simulink model "cesna_a_37_impl"  (Simulink 7.5)
settings: Solver=ode45  StartTime=0.0  StopTime=200  RelTol=1e-3
undefined symbols (not defined in the file): A, alpha_trim, B, C, D, F_T_trim
libraries: simulink x3, Airframes x1
(part 2 of 2)

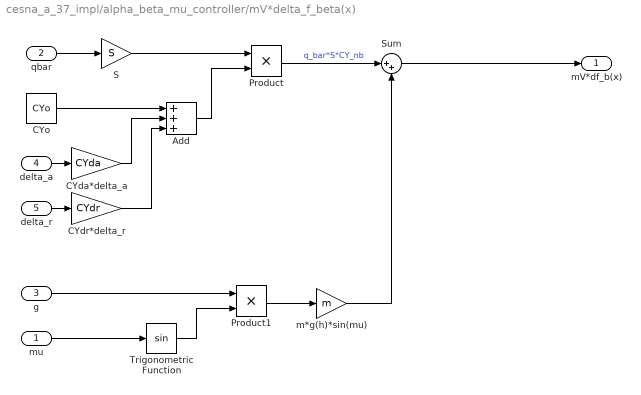
== system cesna_a_37_impl/alpha_beta_mu_controller/mV*delta_f_beta(x) ==
  mu : Inport  OutDataType=fixdt(1, 16)  OutScaling=2^0
  qbar : Inport  Port=2  OutDataType=fixdt(1, 16)  OutScaling=2^0
  g : Inport  Port=3  OutDataType=fixdt(1, 16)  OutScaling=2^0
  delta_a : Inport  Port=4  OutDataType=fixdt(1, 16)  OutScaling=2^0
  delta_r : Inport  Port=5  OutDataType=fixdt(1, 16)  OutScaling=2^0
  Add : Sum  Inputs=+++  OutDataType=fixdt(1, 16)  OutScaling=2^-10
  CYda*delta_a : Gain  Gain=CYda  ParameterDataTypeMode=single  ParameterDataType=fixdt(1, 16)  ParameterScaling=2^0  ParamDataTypeStr=single  OutDataType=fixdt(1, 16)  OutScaling=2^0
  CYdr*delta_r : Gain  Gain=CYdr  ParameterDataTypeMode=single  ParameterDataType=fixdt(1, 16)  ParameterScaling=2^0  ParamDataTypeStr=single  OutDataType=fixdt(1, 16)  OutScaling=2^0
  CYo : Constant  Value=CYo  OutDataTypeMode=single  OutDataType=fixdt(1, 16)  OutScaling=2^0  OutDataTypeStr=single
  Product : Product  OutDataType=fixdt(1, 16)  OutScaling=2^0  RndMeth=Zero
  Product1 : Product  OutDataType=fixdt(1, 16)  OutScaling=2^0  RndMeth=Zero
  S : Gain  Gain=S  ParameterDataTypeMode=single  ParameterDataType=fixdt(1, 16)  ParameterScaling=2^0  ParamDataTypeStr=single  OutDataType=fixdt(1, 16)  OutScaling=2^0
  Sum : Sum  Inputs=|++  OutDataType=fixdt(1, 16)  OutScaling=2^0
  Trigonometric Function : Trigonometry
  m*g(h)*sin(mu) : Gain  Gain=m  ParameterDataTypeMode=single  ParameterDataType=fixdt(1, 16)  ParameterScaling=2^0  ParamDataTypeStr=single  OutDataType=fixdt(1, 16)  OutScaling=2^0
  mV*df_b(x) : Outport  OutDataType=fixdt(1, 16)  OutScaling=2^0
  wires:
  Sum/1 -> mV*df_b(x)/1
  m*g(h)*sin(mu)/1 -> Sum/2
  Product1/1 -> m*g(h)*sin(mu)/1
  Trigonometric Function/1 -> Product1/2
  mu/1 -> Trigonometric Function/1
  g/1 -> Product1/1
  Product/1 -> Sum/1  "q_bar*S*CY_nb"
  CYdr*delta_r/1 -> Add/3
  delta_r/1 -> CYdr*delta_r/1
  delta_a/1 -> CYda*delta_a/1
  CYda*delta_a/1 -> Add/2
  CYo/1 -> Add/1
  Add/1 -> Product/2
  S/1 -> Product/1
  qbar/1 -> S/1

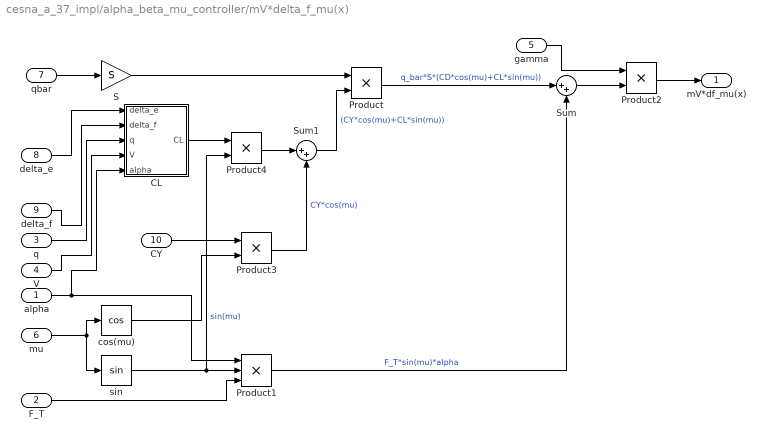
== system cesna_a_37_impl/alpha_beta_mu_controller/mV*delta_f_mu(x) ==
  alpha : Inport  OutDataType=fixdt(1, 16)  OutScaling=2^0
  F_T : Inport  Port=2  OutDataType=fixdt(1, 16)  OutScaling=2^0
  q : Inport  Port=3  OutDataType=fixdt(1, 16)  OutScaling=2^0
  V : Inport  Port=4  OutDataType=fixdt(1, 16)  OutScaling=2^0
  gamma : Inport  Port=5  OutDataType=fixdt(1, 16)  OutScaling=2^0
  mu : Inport  Port=6  OutDataType=fixdt(1, 16)  OutScaling=2^0
  qbar : Inport  Port=7  OutDataType=fixdt(1, 16)  OutScaling=2^0
  delta_e : Inport  Port=8  OutDataType=fixdt(1, 16)  OutScaling=2^0
  delta_f : Inport  Port=9  OutDataType=fixdt(1, 16)  OutScaling=2^0
  CY : Inport  Port=10  OutDataType=fixdt(1, 16)  OutScaling=2^0
  CL : Subsystem
  Product{,2..4} (4 alike) : Product  OutDataType=fixdt(1, 16)  OutScaling=2^0  RndMeth=Zero
  Product1 : Product  Inputs=3  OutDataType=fixdt(1, 16)  OutScaling=2^0  RndMeth=Zero
  S : Gain  Gain=S  ParameterDataTypeMode=single  ParameterDataType=fixdt(1, 16)  ParameterScaling=2^0  ParamDataTypeStr=single  OutDataType=fixdt(1, 16)  OutScaling=2^0
  Sum : Sum  Inputs=|++  OutDataType=fixdt(1, 16)  OutScaling=2^0
  Sum1 : Sum  Inputs=|++  OutDataType=fixdt(1, 16)  OutScaling=2^0
  cos(mu) : Trigonometry  Operator=cos
  sin : Trigonometry
  mV*df_mu(x) : Outport  OutDataType=fixdt(1, 16)  OutScaling=2^0
  wires:
  qbar/1 -> S/1
  S/1 -> Product/1
  Product/1 -> Sum/1  "q_bar*S*(CD*cos(mu)+CL*sin(mu))"
  mu/1 -> sin/1, cos(mu)/1
  Product1/1 -> Sum/2  "F_T*sin(mu)*alpha"
  gamma/1 -> Product2/1
  Sum/1 -> Product2/2
  Product2/1 -> mV*df_mu(x)/1
  F_T/1 -> Product1/3
  sin/1 -> Product1/2, Product4/2  "sin(mu)"
  alpha/1 -> Product1/1, CL/5(alpha)
  delta_f/1 -> CL/2(delta_f)
  delta_e/1 -> CL/1(delta_e)
  Product3/1 -> Sum1/2  "CY*cos(mu)"
  cos(mu)/1 -> Product3/2
  Sum1/1 -> Product/2  "(CY*cos(mu)+CL*sin(mu))"
  q/1 -> CL/3(q)
  V/1 -> CL/4(V)
  CL/1(CL) -> Product4/1
  Product4/1 -> Sum1/1
  CY/1 -> Product3/1

== system cesna_a_37_impl/alpha_beta_mu_controller/sat ==
  mu_set : Inport
  alpha_set : Inport  Port=2
  beta_set : Inport  Port=3
  Mux1 : Mux  Inputs=3
  Saturation1 : Saturate  UpperLimit=pi/4  LowerLimit=-pi/4  OutDataType=fixdt(1, 16)  OutScaling=2^0
  Saturation2 : Saturate  UpperLimit=pi/4  LowerLimit=-pi/4  OutDataType=fixdt(1, 16)  OutScaling=2^0
  Saturation3 : Saturate  UpperLimit=pi/20  LowerLimit=-pi/20  OutDataType=fixdt(1, 16)  OutScaling=2^0
  x_2 : Outport
  wires:
  Mux1/1 -> x_2/1
  mu_set/1 -> Saturation1/1
  alpha_set/1 -> Saturation2/1
  beta_set/1 -> Saturation3/1
  Saturation1/1 -> Mux1/1
  Saturation2/1 -> Mux1/2
  Saturation3/1 -> Mux1/3

== system cesna_a_37_impl/gamma_chi_controller/Calc_CL ==
  alpha : Inport  OutDataType=fixdt(1, 16)  OutScaling=2^0
  delta : Inport  Port=2  OutDataType=fixdt(1, 16)  OutScaling=2^0
  omega : Inport  Port=3  OutDataType=fixdt(1, 16)  OutScaling=2^0
  V : Inport  Port=4  OutDataType=fixdt(1, 16)  OutScaling=2^0
  Add : Sum  Inputs=++++  OutDataType=fixdt(1, 16)  OutScaling=2^-10
  CLa : Gain  Gain=CLa  ParameterDataTypeMode=single  ParameterDataType=fixdt(1, 16)  ParameterScaling=2^0  ParamDataTypeStr=single  OutDataType=fixdt(1, 16)  OutScaling=2^0
  CLo : Constant  Value=CLo  OutDataTypeMode=single  OutDataType=fixdt(1, 16)  OutScaling=2^0  OutDataTypeStr=single
  Divide : Product  Inputs=*/  OutDataType=fixdt(1, 16)  OutScaling=2^-10
  Dot Product : DotProduct  OutDataType=fixdt(1, 16)  OutScaling=2^-10  InputSameDT=on  OutDataTypeStr=Inherit: Inherit via internal rule
  "[CLde,CLin]" : Constant  Value=[CLde,CLin]  OutDataTypeMode=single  OutDataType=fixdt(1, 16)  OutScaling=2^0  OutDataTypeStr=single
  "[q]" : Selector  InputPortWidth=3  IndexOptions=Index vector (dialog)  Indices=[2]  OutputSizes=1
  delta_e,f : Selector  InputPortWidth=4  IndexOptions=Index vector (dialog)  Indices=[1,2]  OutputSizes=1
  q*CLq*cbar/2 : Gain  Gain=CLq*cbar/2  ParameterDataTypeMode=single  ParameterDataType=fixdt(1, 16)  ParameterScaling=2^0  ParamDataTypeStr=single  OutDataType=fixdt(1, 16)  OutScaling=2^0
  CL : Outport  OutDataType=fixdt(1, 16)  OutScaling=2^0
  wires:
  Add/1 -> CL/1
  Divide/1 -> Add/4
  Dot Product/1 -> Add/3
  CLa/1 -> Add/2
  CLo/1 -> Add/1
  V/1 -> Divide/2
  q*CLq*cbar/2/1 -> Divide/1
  alpha/1 -> CLa/1
  "[q]"/1 -> q*CLq*cbar/2/1
  "[CLde,CLin]"/1 -> Dot Product/1
  delta_e,f/1 -> Dot Product/2
  delta/1 -> delta_e,f/1
  omega/1 -> "[q]"/1

== system cesna_a_37_impl/gamma_chi_controller/Calc_CY ==
  beta : Inport  OutDataType=fixdt(1, 16)  OutScaling=2^0
  delta : Inport  Port=2  OutDataType=fixdt(1, 16)  OutScaling=2^0
  omega : Inport  Port=3  OutDataType=fixdt(1, 16)  OutScaling=2^0
  V : Inport  Port=4  OutDataType=fixdt(1, 16)  OutScaling=2^0
  Add : Sum  Inputs=++++  OutDataType=fixdt(1, 16)  OutScaling=2^-10
  CYb : Gain  Gain=CYb  ParameterDataTypeMode=single  ParameterDataType=fixdt(1, 16)  ParameterScaling=2^0  ParamDataTypeStr=single  OutDataType=fixdt(1, 16)  OutScaling=2^0
  CYo : Constant  Value=CYo  OutDataTypeMode=single  OutDataType=fixdt(1, 16)  OutScaling=2^0  OutDataTypeStr=single
  Divide : Product  Inputs=*/  OutDataType=fixdt(1, 16)  OutScaling=2^-10
  Dot Product : DotProduct  OutDataType=fixdt(1, 16)  OutScaling=2^-10  InputSameDT=on  OutDataTypeStr=Inherit: Inherit via internal rule
  Dot Product1 : DotProduct  OutDataType=fixdt(1, 16)  OutScaling=2^-10  InputSameDT=on  OutDataTypeStr=Inherit: Inherit via internal rule
  "[CYda,CYdr]" : Constant  Value=[CYda,CYdr]  OutDataTypeMode=single  OutDataType=fixdt(1, 16)  OutScaling=2^0  OutDataTypeStr=single
  "[CYp,CYr]" : Constant  Value=[CYp,CYr]  OutDataTypeMode=single  OutDataType=fixdt(1, 16)  OutScaling=2^0  OutDataTypeStr=single
  "[p,r]" : Selector  InputPortWidth=3  IndexOptions=Index vector (dialog)  Indices=[1,3]  OutputSizes=1
  b/2 : Gain  Gain=b/2  ParameterDataTypeMode=single  ParameterDataType=fixdt(1, 16)  ParameterScaling=2^0  ParamDataTypeStr=single  OutDataType=fixdt(1, 16)  OutScaling=2^0
  delta_a,r : Selector  InputPortWidth=4  IndexOptions=Index vector (dialog)  Indices=[3,4]  OutputSizes=1
  CY : Outport  OutDataType=fixdt(1, 16)  OutScaling=2^0
  wires:
  omega/1 -> "[p,r]"/1
  delta/1 -> delta_a,r/1
  delta_a,r/1 -> Dot Product/2
  "[CYda,CYdr]"/1 -> Dot Product/1
  "[CYp,CYr]"/1 -> Dot Product1/1
  "[p,r]"/1 -> Dot Product1/2
  beta/1 -> CYb/1
  Dot Product1/1 -> b/2/1
  b/2/1 -> Divide/1
  V/1 -> Divide/2
  CYo/1 -> Add/1
  CYb/1 -> Add/2
  Dot Product/1 -> Add/3
  Divide/1 -> Add/4
  Add/1 -> CY/1

== system cesna_a_37_impl/gamma_chi_controller/Hz_ipesh ==
  u : Inport
  Discrete State-Space : DiscreteStateSpace  A=A  B=B  C=C  D=D  X0=x0  SampleTime=Ts
  y : Outport
  wires:
  u/1 -> Discrete State-Space/1
  Discrete State-Space/1 -> y/1

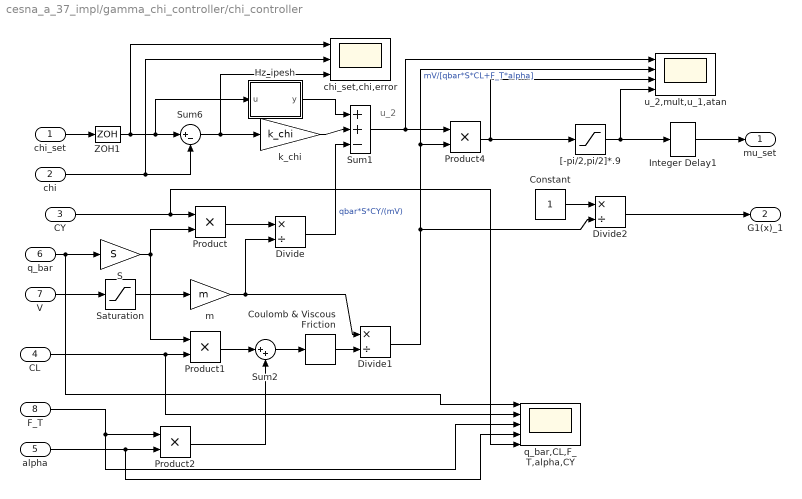
== system cesna_a_37_impl/gamma_chi_controller/chi_controller ==
  note: u_2
  chi_set : Inport
  chi : Inport  Port=2
  CY : Inport  Port=3
  CL : Inport  Port=4
  alpha : Inport  Port=5
  q_bar : Inport  Port=6
  V : Inport  Port=7
  F_T : Inport  Port=8
  Constant : Constant  OutDataTypeMode=single  OutDataType=fixdt(1, 16)  OutScaling=2^0  OutDataTypeStr=single
  Coulomb & Viscous Friction : simulink/Discontinuities/Coulomb & Viscous Friction  SystemSampleTime=-1  offset=.01  gain=1
  Divide : Product  Inputs=*/  OutDataType=fixdt(1, 16)  OutScaling=2^-10
  Divide1 : Product  Inputs=*/  OutDataType=fixdt(1, 16)  OutScaling=2^-10
  Divide2 : Product  Inputs=*/  OutDataType=fixdt(1, 16)  OutScaling=2^-10
  Hz_ipesh : Subsystem  mask{num=[1,0], den=[10*Ts/pi,1], Ts=Ts, y0=0}
      mask prompts: num "Hs num [num]"; den "Hs den [den]"; Ts "Sample Period (s) [Ts]"; y0 "y0 (N)"
      mask init:
      | Hs=tf(num,den);
      | Hz=ipesh_transform(Hs,Ts);
      | [A,B,C,D]=tf2ss(Hz.num{1},Hz.den{1});
      | x0=y0/C;
  Integer Delay1 : simulink/Discrete/Integer Delay  vinit=0.0  samptime=-1  NumDelays=1
  Product{,1..2,4} (4 alike) : Product  OutDataType=fixdt(1, 16)  OutScaling=2^0  RndMeth=Zero
  S : Gain  Gain=S  ParameterDataTypeMode=single  ParameterDataType=fixdt(1, 16)  ParameterScaling=2^0  ParamDataTypeStr=single  OutDataType=fixdt(1, 16)  OutScaling=2^0
  Saturation : Saturate  UpperLimit=inf  LowerLimit=10  OutDataType=fixdt(1, 16)  OutScaling=2^0
  Sum1 : Sum  Inputs=|++-  OutDataType=fixdt(1, 16)  OutScaling=2^0
  Sum2 : Sum  Inputs=|++  OutDataType=fixdt(1, 16)  OutScaling=2^0
  Sum6 : Sum  Inputs=|+-  OutDataType=fixdt(1, 16)  OutScaling=2^0
  ZOH1 : ZeroOrderHold  SampleTime=Ts
  "[-pi/2,pi/2]*.9" : Saturate  UpperLimit=.9*pi/2  LowerLimit=-.9*pi/2  OutDataType=fixdt(1, 16)  OutScaling=2^0
  chi_set,chi,error : Scope  NumInputPorts=3
      settings: YMin=0~-0.05~-0.0075  YMax=0.5~0.55~0.02  SaveName=chi_s  SampleInput=on  SampleTime=0.05
  k_chi : Gain  Gain=k_chi  ParameterDataTypeMode=single  ParameterDataType=fixdt(1, 16)  ParameterScaling=2^0  ParamDataTypeStr=single  OutDataType=fixdt(1, 16)  OutScaling=2^0
  m : Gain  Gain=m  ParameterDataTypeMode=single  ParameterDataType=fixdt(1, 16)  ParameterScaling=2^0  ParamDataTypeStr=single  OutDataType=fixdt(1, 16)  OutScaling=2^0
  q_bar,CL,F_T,alpha,CY : Scope  NumInputPorts=5
      settings: YMin=9000~0.1~0~-0.025~-0.035  YMax=12500~0.23~25000~0.005~0.005  SaveName=ScopeData11  SampleInput=on  SampleTime=0.05
  u_2,mult,u_1,atan : Scope  NumInputPorts=4
      settings: YMin=-0.001~9.7~-0.01~-0.01  YMax=0.003~11~0.03~0.03  SaveName=ScopeData8  SampleInput=on  SampleTime=0.04
  mu_set : Outport
  G1(x)_1 : Outport  Port=2
  wires:
  Sum6/1 -> k_chi/1, chi_set,chi,error/3
  ZOH1/1 -> chi_set,chi,error/1, Sum6/1, Hz_ipesh/1(u)
  chi_set/1 -> ZOH1/1
  chi/1 -> Sum6/2, chi_set,chi,error/2
  CY/1 -> Product/1, q_bar,CL,F_T,alpha,CY/5
  q_bar/1 -> S/1, q_bar,CL,F_T,alpha,CY/1
  V/1 -> Saturation/1
  m/1 -> Divide/2, Divide1/1
  S/1 -> Product/2, Product1/1
  Product/1 -> Divide/1
  alpha/1 -> Product2/2, q_bar,CL,F_T,alpha,CY/4
  Product1/1 -> Sum2/1
  Sum2/1 -> Coulomb & Viscous Friction/1
  Sum1/1 -> Product4/1, u_2,mult,u_1,atan/1
  Divide1/1 -> Product4/2, u_2,mult,u_1,atan/2, Divide2/2  "mV/[qbar*S*CL+F_T*alpha]"
  Product4/1 -> u_2,mult,u_1,atan/3, "[-pi/2,pi/2]*.9"/1
  "[-pi/2,pi/2]*.9"/1 -> Integer Delay1/1, u_2,mult,u_1,atan/4
  Coulomb & Viscous Friction/1 -> Divide1/2
  Saturation/1 -> m/1
  CL/1 -> Product1/2, q_bar,CL,F_T,alpha,CY/2
  F_T/1 -> Product2/1, q_bar,CL,F_T,alpha,CY/3
  Product2/1 -> Sum2/2
  Integer Delay1/1 -> mu_set/1
  k_chi/1 -> Sum1/2
  Divide/1 -> Sum1/3  "qbar*S*CY/(mV)"
  Hz_ipesh/1(y) -> Sum1/1
  Divide2/1 -> G1(x)_1/1
  Constant/1 -> Divide2/1

== system cesna_a_37_impl/gamma_chi_mu_sensor/calc_chi ==
  v_I1 : Inport
  v_I2 : Inport  Port=2
  Divide : Product  Inputs=*/  OutDataType=fixdt(1, 16)  OutScaling=2^-10
  Dot Product : DotProduct  OutDataType=fixdt(1, 16)  OutScaling=2^-10  InputSameDT=on  OutDataTypeStr=Inherit: Inherit via internal rule
  Math Function : Math  Operator=sqrt  OutDataType=fixdt(1, 16)  OutScaling=2^0  SaturateOnIntegerOverflow=on
  Mux : Mux  Inputs=2
  asin : Trigonometry  Operator=asin
  chi : Outport
  wires:
  v_I1/1 -> Mux/1
  v_I2/1 -> Mux/2, Divide/1
  Mux/1 -> Dot Product/1, Dot Product/2
  Dot Product/1 -> Math Function/1
  Math Function/1 -> Divide/2
  Divide/1 -> asin/1
  asin/1 -> chi/1

== system cesna_a_37_impl/gamma_chi_mu_sensor/calc_gamma ==
  v_I3 : Inport
  V : Inport  Port=2
  Divide : Product  Inputs=*/  OutDataType=fixdt(1, 16)  OutScaling=2^-10
  Gain : Gain  Gain=-1  ParameterDataTypeMode=single  ParameterDataType=fixdt(1, 16)  ParameterScaling=2^0  ParamDataTypeStr=single  OutDataType=fixdt(1, 16)  OutScaling=2^0
  Trigonometric Function : Trigonometry  Operator=asin
  gamma : Outport
  wires:
  Divide/1 -> Gain/1
  Gain/1 -> Trigonometric Function/1
  v_I3/1 -> Divide/1
  Trigonometric Function/1 -> gamma/1
  V/1 -> Divide/2

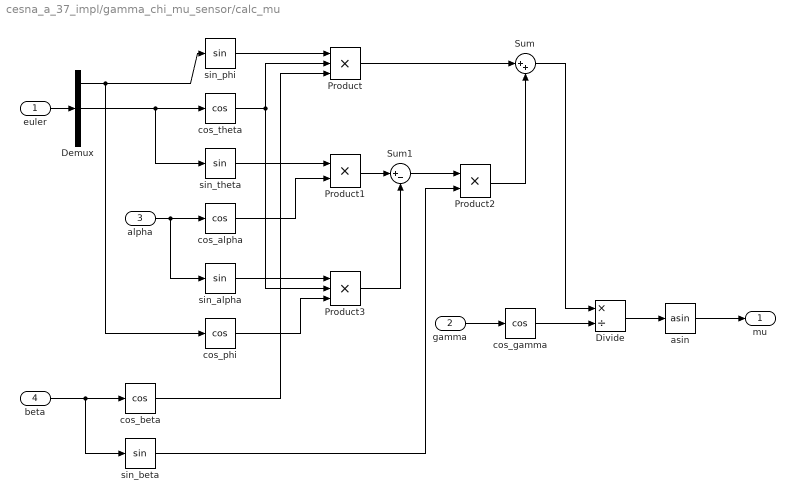
== system cesna_a_37_impl/gamma_chi_mu_sensor/calc_mu ==
  euler : Inport
  gamma : Inport  Port=2
  alpha : Inport  Port=3
  beta : Inport  Port=4
  Demux : Demux  Outputs=3
  Divide : Product  Inputs=*/  OutDataType=fixdt(1, 16)  OutScaling=2^-10
  Product : Product  Inputs=3  OutDataType=fixdt(1, 16)  OutScaling=2^0  RndMeth=Zero
  Product1 : Product  OutDataType=fixdt(1, 16)  OutScaling=2^0  RndMeth=Zero
  Product2 : Product  OutDataType=fixdt(1, 16)  OutScaling=2^0  RndMeth=Zero
  Product3 : Product  Inputs=3  OutDataType=fixdt(1, 16)  OutScaling=2^0  RndMeth=Zero
  Sum : Sum  Inputs=|++  OutDataType=fixdt(1, 16)  OutScaling=2^0
  Sum1 : Sum  Inputs=|+-  OutDataType=fixdt(1, 16)  OutScaling=2^0
  asin : Trigonometry  Operator=asin
  cos_alpha : Trigonometry  Operator=cos
  cos_beta : Trigonometry  Operator=cos
  cos_gamma : Trigonometry  Operator=cos
  cos_phi : Trigonometry  Operator=cos
  cos_theta : Trigonometry  Operator=cos
  sin_alpha : Trigonometry
  sin_beta : Trigonometry
  sin_phi : Trigonometry
  sin_theta : Trigonometry
  mu : Outport
  wires:
  gamma/1 -> cos_gamma/1
  cos_gamma/1 -> Divide/2
  Divide/1 -> asin/1
  euler/1 -> Demux/1
  alpha/1 -> cos_alpha/1, sin_alpha/1
  Demux/2 -> cos_theta/1, sin_theta/1
  Demux/1 -> sin_phi/1, cos_phi/1
  sin_phi/1 -> Product/1
  cos_theta/1 -> Product/2, Product3/2
  sin_theta/1 -> Product1/1
  Product/1 -> Sum/1
  Sum/1 -> Divide/1
  beta/1 -> cos_beta/1, sin_beta/1
  cos_beta/1 -> Product/3
  cos_alpha/1 -> Product1/2
  asin/1 -> mu/1
  Product1/1 -> Sum1/1
  Sum1/1 -> Product2/1
  sin_beta/1 -> Product2/2
  sin_alpha/1 -> Product3/1
  cos_phi/1 -> Product3/3
  Product3/1 -> Sum1/2
  Product2/1 -> Sum/2

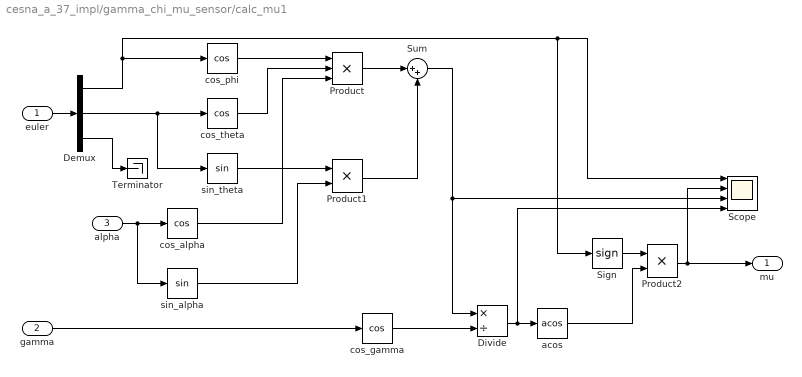
== system cesna_a_37_impl/gamma_chi_mu_sensor/calc_mu1 ==
  euler : Inport
  gamma : Inport  Port=2
  alpha : Inport  Port=3
  Demux : Demux  Outputs=3
  Divide : Product  Inputs=*/  OutDataType=fixdt(1, 16)  OutScaling=2^-10
  Product : Product  Inputs=3  OutDataType=fixdt(1, 16)  OutScaling=2^0  RndMeth=Zero
  Product1 : Product  OutDataType=fixdt(1, 16)  OutScaling=2^0  RndMeth=Zero
  Product2 : Product  OutDataType=fixdt(1, 16)  OutScaling=2^0  RndMeth=Zero
  Scope : Scope  NumInputPorts=4
      settings: YMin=-5~-5~-5~-5  YMax=5~5~5~5  SaveName=ScopeData6  SampleInput=on  SampleTime=.01
  Sign : Signum
  Sum : Sum  Inputs=|++  OutDataType=fixdt(1, 16)  OutScaling=2^0
  Terminator : Terminator
  acos : Trigonometry  Operator=acos
  cos_alpha : Trigonometry  Operator=cos
  cos_gamma : Trigonometry  Operator=cos
  cos_phi : Trigonometry  Operator=cos
  cos_theta : Trigonometry  Operator=cos
  sin_alpha : Trigonometry
  sin_theta : Trigonometry
  mu : Outport
  wires:
  Product2/1 -> Scope/2, mu/1
  acos/1 -> Product2/2
  Sign/1 -> Product2/1
  Sum/1 -> Scope/3, Divide/1
  Product1/1 -> Sum/2
  Product/1 -> Sum/1
  sin_alpha/1 -> Product1/2
  sin_theta/1 -> Product1/1
  cos_alpha/1 -> Product/3
  cos_theta/1 -> Product/2
  cos_phi/1 -> Product/1
  Demux/3 -> Terminator/1
  Demux/1 -> Sign/1, Scope/1, cos_phi/1
  Demux/2 -> sin_theta/1, cos_theta/1
  alpha/1 -> sin_alpha/1, cos_alpha/1
  euler/1 -> Demux/1
  Divide/1 -> Scope/4, acos/1
  cos_gamma/1 -> Divide/2
  gamma/1 -> cos_gamma/1

== system cesna_a_37_impl/gamma_chi_mu_sensor/gravity model ==
  h : Inport
  Divide : Product  Inputs=*/  OutDataType=fixdt(1, 16)  OutScaling=2^-10
  Dot Product1 : DotProduct  OutDataType=fixdt(1, 16)  OutScaling=2^-10  InputSameDT=on  OutDataTypeStr=Inherit: Inherit via internal rule
  Model Info : simulink/Model-Wide Utilities/Model Info  SystemSampleTime=-1  InitialBlockCM=None  BlockCM=None  Frame=on  DisplayStringWithTags=g = g_o [R/(R+h)]^2  HorizontalTextAlignment=Center  LeftAlignmentValue=0.5  SourceBlockDiagram=cesna_a_37_impl  TagMaxNumber=20
  R = Radius of Earth (m) : Constant  Value=6356e3  OutDataTypeMode=single  OutDataType=fixdt(1, 16)  OutScaling=2^0  OutDataTypeStr=single  SampleTime=Ts
  Sum : Sum  Inputs=|++  OutDataType=fixdt(1, 16)  OutScaling=2^0
  g_o : Gain  Gain=9.80665  ParameterDataTypeMode=single  ParameterDataType=fixdt(1, 16)  ParameterScaling=2^0  ParamDataTypeStr=single  OutDataType=fixdt(1, 16)  OutScaling=2^0
  g : Outport
  wires:
  g_o/1 -> g/1
  h/1 -> Sum/1
  Dot Product1/1 -> g_o/1
  Divide/1 -> Dot Product1/2, Dot Product1/1
  Sum/1 -> Divide/2
  R = Radius of Earth (m)/1 -> Divide/1, Sum/2

== system cesna_a_37_impl/omega_controller/alg_loop_filt ==
  u : Inport
  Demux : Demux  Outputs=3
  Hz_ipesh : Subsystem  mask{num=[1], den=[10*Ts/pi,1], Ts=Ts, y0=0}
      mask prompts: num "Hs num [num]"; den "Hs den [den]"; Ts "Sample Period (s) [Ts]"; y0 "y0 (N)"
      mask init:
      | Hs=tf(num,den);
      | Hz=ipesh_transform(Hs,Ts);
      | [A,B,C,D]=tf2ss(Hz.num{1},Hz.den{1});
      | x0=y0/C;
  Hz_ipesh1 : Subsystem  mask{num=[1,0], den=[10*Ts/pi,1], Ts=Ts, y0=0}
      mask prompts: num "Hs num [num]"; den "Hs den [den]"; Ts "Sample Period (s) [Ts]"; y0 "y0 (N)"
      mask init:
      | Hs=tf(num,den);
      | Hz=ipesh_transform(Hs,Ts);
      | [A,B,C,D]=tf2ss(Hz.num{1},Hz.den{1});
      | x0=y0/C;
  Hz_ipesh2 : Subsystem  mask{num=[1,0], den=[10*Ts/pi,1], Ts=Ts, y0=0}
      mask prompts: num "Hs num [num]"; den "Hs den [den]"; Ts "Sample Period (s) [Ts]"; y0 "y0 (N)"
      mask init:
      | Hs=tf(num,den);
      | Hz=ipesh_transform(Hs,Ts);
      | [A,B,C,D]=tf2ss(Hz.num{1},Hz.den{1});
      | x0=y0/C;
  Mux2 : Mux  Inputs=3
  y : Outport
  wires:
  u/1 -> Demux/1
  Demux/1 -> Hz_ipesh/1(u)
  Hz_ipesh/1(y) -> Mux2/1
  Demux/2 -> Hz_ipesh1/1(u)
  Hz_ipesh1/1(y) -> Mux2/2
  Demux/3 -> Hz_ipesh2/1(u)
  Hz_ipesh2/1(y) -> Mux2/3
  Mux2/1 -> y/1

== system cesna_a_37_impl/omega_controller/omega_set_dot ==
  omega_set : Inport
  Demux : Demux  Outputs=3
  Hz_ipesh : Subsystem  mask{num=[1,0], den=[10*Ts/pi,1], Ts=Ts, y0=0}
      mask prompts: num "Hs num [num]"; den "Hs den [den]"; Ts "Sample Period (s) [Ts]"; y0 "y0 (N)"
      mask init:
      | Hs=tf(num,den);
      | Hz=ipesh_transform(Hs,Ts);
      | [A,B,C,D]=tf2ss(Hz.num{1},Hz.den{1});
      | x0=y0/C;
  Hz_ipesh1 : Subsystem  mask{num=[1,0], den=[10*Ts/pi,1], Ts=Ts, y0=0}
      mask prompts: num "Hs num [num]"; den "Hs den [den]"; Ts "Sample Period (s) [Ts]"; y0 "y0 (N)"
      mask init:
      | Hs=tf(num,den);
      | Hz=ipesh_transform(Hs,Ts);
      | [A,B,C,D]=tf2ss(Hz.num{1},Hz.den{1});
      | x0=y0/C;
  Hz_ipesh2 : Subsystem  mask{num=[1,0], den=[10*Ts/pi,1], Ts=Ts, y0=0}
      mask prompts: num "Hs num [num]"; den "Hs den [den]"; Ts "Sample Period (s) [Ts]"; y0 "y0 (N)"
      mask init:
      | Hs=tf(num,den);
      | Hz=ipesh_transform(Hs,Ts);
      | [A,B,C,D]=tf2ss(Hz.num{1},Hz.den{1});
      | x0=y0/C;
  Mux2 : Mux  Inputs=3
  omega_set_dot : Outport
  wires:
  omega_set/1 -> Demux/1
  Demux/1 -> Hz_ipesh/1(u)
  Hz_ipesh/1(y) -> Mux2/1
  Demux/2 -> Hz_ipesh1/1(u)
  Hz_ipesh1/1(y) -> Mux2/2
  Demux/3 -> Hz_ipesh2/1(u)
  Hz_ipesh2/1(y) -> Mux2/3
  Mux2/1 -> omega_set_dot/1

== system cesna_a_37_impl/velocity_controller/Dynamic Pressure ==
  V : Inport  OutDataType=sfix(16)  OutScaling=2^0
  Air Density : Inport  Port=2  OutDataType=sfix(16)  OutScaling=2^0
  1/2rhoV^2 : Gain  Gain=1/2  ParameterDataTypeMode=single  ParameterDataType=sfix(16)  ParameterScaling=2^0  ParamDataTypeStr=single  OutDataType=sfix(16)  OutScaling=2^0  SaturateOnIntegerOverflow=on  OutDataTypeStr=Inherit: Same as input
  Product1 : Product  OutDataType=sfix(16)  OutScaling=2^0  SaturateOnIntegerOverflow=on  InputSameDT=on  OutDataTypeStr=Inherit: Same as first input
  Product2 : Product  OutDataType=sfix(16)  OutScaling=2^0  SaturateOnIntegerOverflow=on  InputSameDT=on  OutDataTypeStr=Inherit: Same as first input
  qbar : Outport  OutDataType=sfix(16)  OutScaling=2^0  InitialOutput=0
  wires:
  1/2rhoV^2/1 -> qbar/1
  Product2/1 -> 1/2rhoV^2/1
  Air Density/1 -> Product2/2
  Product1/1 -> Product2/1
  V/1 -> Product1/1, Product1/2

== system cesna_a_37_impl/velocity_controller/Hz_ipesh ==
  u : Inport
  Discrete State-Space : DiscreteStateSpace  A=A  B=B  C=C  D=D  X0=x0  SampleTime=Ts
  y : Outport
  wires:
  u/1 -> Discrete State-Space/1
  Discrete State-Space/1 -> y/1

== system cesna_a_37_impl/velocity_controller/Vs_filt ==
  u : Inport
  Discrete State-Space : DiscreteStateSpace  A=A  B=B  C=C  D=D  X0=x0  SampleTime=Ts
  y : Outport
  wires:
  Discrete State-Space/1 -> y/1
  u/1 -> Discrete State-Space/1

== system cesna_a_37_impl/velocity_controller/anti_windup_control ==
  In1 : Inport
  Add4 : Sum  Inputs=+-  OutDataType=fixdt(1, 16)  OutScaling=2^-10
  Hz_ideal_plant : Subsystem  mask{num=[1], den=m*[1,omega_d], Ts=Ts, y0=0}
      mask prompts: num "Hs num [num]"; den "Hs den [den]"; Ts "Sample Period (s) [Ts]"; y0 "y0 (N)"
      mask init:
      | Hs=tf(num,den);
      | Hz=ipesh_transform(Hs,Ts);
      | [A,B,C,D]=tf2ss(Hz.num{1},Hz.den{1});
      | x0=y0/C;
  Saturation : Saturate  UpperLimit=inf  LowerLimit=0  OutDataType=fixdt(1, 16)  OutScaling=2^0
  Out1 : Outport
  Out2 : Outport  Port=2
  wires:
  In1/1 -> Add4/1, Saturation/1
  Saturation/1 -> Add4/2, Out1/1
  Add4/1 -> Hz_ideal_plant/1(u)
  Hz_ideal_plant/1(y) -> Out2/1

== system cesna_a_37_impl/alpha_beta_mu_controller/alg_loop_filt/Hz_ipesh ==
  u : Inport
  Discrete State-Space : DiscreteStateSpace  A=A  B=B  C=C  D=D  X0=x0  SampleTime=Ts
  y : Outport
  wires:
  u/1 -> Discrete State-Space/1
  Discrete State-Space/1 -> y/1

== system cesna_a_37_impl/alpha_beta_mu_controller/alg_loop_filt/Hz_ipesh1 ==
  u : Inport
  Discrete State-Space : DiscreteStateSpace  A=A  B=B  C=C  D=D  X0=x0  SampleTime=Ts
  y : Outport
  wires:
  Discrete State-Space/1 -> y/1
  u/1 -> Discrete State-Space/1

== system cesna_a_37_impl/alpha_beta_mu_controller/alg_loop_filt/Hz_ipesh2 ==
  u : Inport
  Discrete State-Space : DiscreteStateSpace  A=A  B=B  C=C  D=D  X0=x0  SampleTime=Ts
  y : Outport
  wires:
  u/1 -> Discrete State-Space/1
  Discrete State-Space/1 -> y/1

== system cesna_a_37_impl/alpha_beta_mu_controller/mV*delta_f_mu(x)/CL ==
  delta_e : Inport  OutDataType=fixdt(1, 16)  OutScaling=2^0
  delta_f : Inport  Port=2  OutDataType=fixdt(1, 16)  OutScaling=2^0
  q : Inport  Port=3  OutDataType=fixdt(1, 16)  OutScaling=2^0
  V : Inport  Port=4  OutDataType=fixdt(1, 16)  OutScaling=2^0
  alpha : Inport  Port=5  OutDataType=fixdt(1, 16)  OutScaling=2^0
  Add : Sum  Inputs=+++++  OutDataType=fixdt(1, 16)  OutScaling=2^-10
  CDo : Constant  Value=CLo  OutDataTypeMode=single  OutDataType=fixdt(1, 16)  OutScaling=2^0  OutDataTypeStr=single
  CLa*alpha : Gain  Gain=CLa  ParameterDataTypeMode=single  ParameterDataType=fixdt(1, 16)  ParameterScaling=2^0  ParamDataTypeStr=single  OutDataType=fixdt(1, 16)  OutScaling=2^0
  CLde*delta_e : Gain  Gain=CLde  ParameterDataTypeMode=single  ParameterDataType=fixdt(1, 16)  ParameterScaling=2^0  ParamDataTypeStr=single  OutDataType=fixdt(1, 16)  OutScaling=2^0
  CLin*delta_f : Gain  Gain=CLin  ParameterDataTypeMode=single  ParameterDataType=fixdt(1, 16)  ParameterScaling=2^0  ParamDataTypeStr=single  OutDataType=fixdt(1, 16)  OutScaling=2^0
  Divide : Product  Inputs=*/  OutDataType=fixdt(1, 16)  OutScaling=2^-10
  q*cbar*CLq/2 : Gain  Gain=cbar*CLq/2  ParameterDataTypeMode=single  ParameterDataType=fixdt(1, 16)  ParameterScaling=2^0  ParamDataTypeStr=single  OutDataType=fixdt(1, 16)  OutScaling=2^0
  CL : Outport
  wires:
  Divide/1 -> Add/5
  V/1 -> Divide/2
  q*cbar*CLq/2/1 -> Divide/1
  q/1 -> q*cbar*CLq/2/1
  CLa*alpha/1 -> Add/4
  CLin*delta_f/1 -> Add/3
  delta_f/1 -> CLin*delta_f/1
  Add/1 -> CL/1
  alpha/1 -> CLa*alpha/1
  delta_e/1 -> CLde*delta_e/1
  CLde*delta_e/1 -> Add/2
  CDo/1 -> Add/1

== system cesna_a_37_impl/gamma_chi_controller/chi_controller/Hz_ipesh ==
  u : Inport
  Discrete State-Space : DiscreteStateSpace  A=A  B=B  C=C  D=D  X0=x0  SampleTime=Ts
  y : Outport
  wires:
  Discrete State-Space/1 -> y/1
  u/1 -> Discrete State-Space/1

== system cesna_a_37_impl/omega_controller/alg_loop_filt/Hz_ipesh ==
  u : Inport
  Discrete State-Space : DiscreteStateSpace  A=A  B=B  C=C  D=D  X0=x0  SampleTime=Ts
  y : Outport
  wires:
  Discrete State-Space/1 -> y/1
  u/1 -> Discrete State-Space/1

== system cesna_a_37_impl/omega_controller/alg_loop_filt/Hz_ipesh1 ==
  u : Inport
  Discrete State-Space : DiscreteStateSpace  A=A  B=B  C=C  D=D  X0=x0  SampleTime=Ts
  y : Outport
  wires:
  u/1 -> Discrete State-Space/1
  Discrete State-Space/1 -> y/1

== system cesna_a_37_impl/omega_controller/alg_loop_filt/Hz_ipesh2 ==
  u : Inport
  Discrete State-Space : DiscreteStateSpace  A=A  B=B  C=C  D=D  X0=x0  SampleTime=Ts
  y : Outport
  wires:
  Discrete State-Space/1 -> y/1
  u/1 -> Discrete State-Space/1

== system cesna_a_37_impl/omega_controller/omega_set_dot/Hz_ipesh ==
  u : Inport
  Discrete State-Space : DiscreteStateSpace  A=A  B=B  C=C  D=D  X0=x0  SampleTime=Ts
  y : Outport
  wires:
  Discrete State-Space/1 -> y/1
  u/1 -> Discrete State-Space/1

== system cesna_a_37_impl/omega_controller/omega_set_dot/Hz_ipesh1 ==
  u : Inport
  Discrete State-Space : DiscreteStateSpace  A=A  B=B  C=C  D=D  X0=x0  SampleTime=Ts
  y : Outport
  wires:
  u/1 -> Discrete State-Space/1
  Discrete State-Space/1 -> y/1

== system cesna_a_37_impl/omega_controller/omega_set_dot/Hz_ipesh2 ==
  u : Inport
  Discrete State-Space : DiscreteStateSpace  A=A  B=B  C=C  D=D  X0=x0  SampleTime=Ts
  y : Outport
  wires:
  Discrete State-Space/1 -> y/1
  u/1 -> Discrete State-Space/1

== system cesna_a_37_impl/velocity_controller/anti_windup_control/Hz_ideal_plant ==
  u : Inport
  Discrete State-Space : DiscreteStateSpace  A=A  B=B  C=C  D=D  X0=x0  SampleTime=Ts
  y : Outport
  wires:
  Discrete State-Space/1 -> y/1
  u/1 -> Discrete State-Space/1

== matlab function alpha_beta_mu_controller/G_2_inverse ==
  settings: updateMethod=DISCRETE  sampleTime=Ts
  data: e input double; omega_d output double; alpha input double; rho input double; CLq parameter double; cbar parameter double; m parameter double; b parameter double; CYp parameter double; CYr parameter double; hat_x2 input double; G2_T_hat_x2 output double
function [omega_d,G2_T_hat_x2] = fcn(e, alpha, rho, CLq, cbar, m, b, CYp, CYr, hat_x2)
%#eml
c_22=1-(rho*CLq*cbar/(4*m));
c_31=(alpha+(b*rho*CYp/(4*m)));
c_33=-1+(b*rho*CYr/(4*m));
den=c_33 - (alpha*c_31);
G2_i=[c_33/den,0,-alpha/den;0,1/c_22,0;-c_31/den,0,1/den];
omega_d = G2_i*e;
G2=[1,0,alpha;0,c_22,0;c_31,0,c_33];
G2_T_hat_x2=G2' * hat_x2;

== matlab function gamma_chi_mu_sensor/Air Properties ==
  data: h input double; T output double; rho output double; g input double; ps output double; a output double
function [T,rho, ps, a] = fcn(h, g)
    %h altitude (meters)
    %g gravity at h (m/s^2)
    R = 8.31432; %J/(mol-Kelvin)
    M = 28.9644; %gm/mol
    To = 288.15; %standard temperature [Kelvin]
    Po = 101325; %standard pressure [Pa]
    L = 6.5; %Kelvin/km
    gamma = 1.4; %Gas constant for air
    T = To - 1.0e-3*L*h;            %Temperature at h
    ps = Po*(T/To)^((g*M)/(R*L));   %Pressure at h
    rho = ps/((1000*R/M)*T);        %Density at h
    a = sqrt(gamma*(R/(M*1e-3))*T); %speed of sound (m/s)

== matlab function omega_controller/Gamma_omega ==
  data: q_bar input double; Gamma_omega output double; omega input double; Clp parameter double; Clr parameter double; Cmq parameter double; Cnp parameter double; Cnr parameter double; S parameter double; b parameter double; cbar parameter double; V input double
function Gamma_omega = fcn(q_bar, omega, Clp, Clr, Cmq, Cnp, Cnr, S, b, cbar, V)
Gamma_omega=0*omega;
p=omega(1);
q=omega(2);
r=omega(3);
temp=q_bar*S/(2*V);
Gamma_omega(1)=temp*b*b*(Clp*p+Clr*r);
Gamma_omega(2)=temp*cbar*cbar*Cmq*q;
Gamma_omega(3)=temp*b*b*(Cnp*p+Cnr*r);
